simulink model "kinematics_ellipse"  (R2015a)
settings: Solver=ode45  StartTime=0.0  StopTime=500  RelTol=1e-3
libraries: simulink x1
settings Model: Creator=MCLab  LastModifiedBy=MCLab

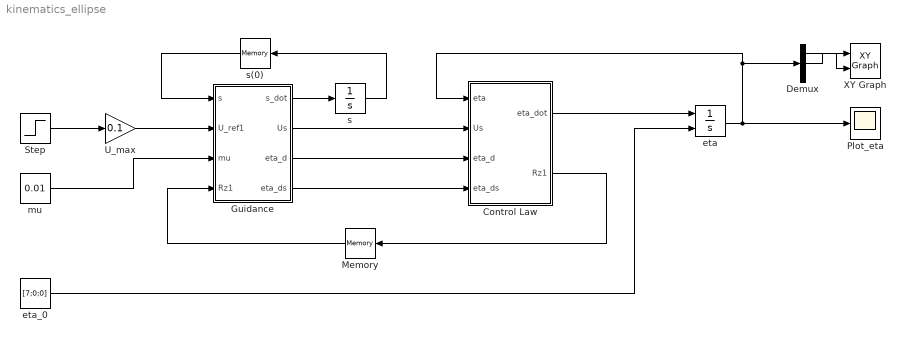
== system kinematics_ellipse ==
  Control Law : MATLAB Function  TreatAsAtomicUnit=on
  Demux : Demux  Outputs=3
  Guidance : MATLAB Function  TreatAsAtomicUnit=on
  Memory : Memory  X0=[0;0;0]
  Plot_eta : Scope
  Step : Step  Time=2000  Before=1  After=-1  SampleTime=0
  U_max : Gain  Gain=0.1
  XY Graph : simulink/Sinks/XY Graph  xmin=-15  xmax=15  ymin=-15  ymax=15  st=-1
  eta : Integrator  InitialConditionSource=external
  eta_0 : Constant  Value=[7;0;0]
  mu : Constant  Value=0.01
  s : Integrator
  s(0) : Memory
  wires:
  Step/1 -> U_max/1
  U_max/1 -> Guidance/2(U_ref1)
  mu/1 -> Guidance/3(mu)
  Guidance/1(s_dot) -> s/1
  s/1 -> s(0)/1
  Guidance/3(eta_d) -> Control Law/3(eta_d)
  Guidance/4(eta_ds) -> Control Law/4(eta_ds)
  Control Law/1(eta_dot) -> eta/1
  eta_0/1 -> eta/2
  Control Law/2(Rz1) -> Memory/1
  Memory/1 -> Guidance/4(Rz1)
  eta/1 -> Plot_eta/1, Control Law/1(eta), Demux/1
  Guidance/2(Us) -> Control Law/2(Us)
  Demux/1 -> XY Graph/2
  Demux/2 -> XY Graph/1
  s(0)/1 -> Guidance/1(s)

== matlab function kinematics_ellipse/Guidance ==
  data: s input; s_dot output; Us output; U_ref1 input; mu input; Rz1 input; eta_d output; eta_ds output
function [s_dot,Us,eta_d,eta_ds] = f(s,U_ref1,mu,Rz1)

%% Ellipse Kinematics

eta_d = [0;0;0];
eta_ds = [0;0;0];

cx = 6;
cy = 0;
rx = 5;
ry = 3;

x_d = cx+rx*cos(s);
y_d = cy+ry*sin(s);

x_ds = -rx*sin(s);
y_ds = ry*cos(s);

x_ds2 = -rx*cos(s);
y_ds2 = -ry*sin(s);

x_ds3 = rx*sin(s);
y_ds3 = -ry*cos(s);

psi_d = atan2(y_ds,x_ds);
psi_ds = (-y_ds*x_ds+x_ds*y_ds2)/(x_ds^2+y_ds^2);
psi_ds2 = ( (-y_ds*x_ds3+x_ds*y_ds3)*(x_ds^2+y_ds^2) - (-y_ds*x_ds2+x_ds*y_ds2)*(2*x_ds2*x_ds+2*y_ds2*y_ds) )/(x_ds^2+y_ds^2)^2;

eta_d = [x_d;y_d;psi_d] ;
eta_ds = [x_ds;y_ds;psi_ds];
eta_ds2 = [x_ds2;y_ds2;psi_ds2];

U_ref2 = U_ref1 ;
Us = U_ref1 / (x_ds^2+y_ds^2)^(1/2);
Us_s = U_ref1 * (x_ds*x_ds2 + y_ds*y_ds2) / (x_ds^2+y_ds^2)^(3/2);


%% Update Law

V1 = - eta_ds'*Rz1 ;
s_dot = Us - mu*V1/norm(eta_ds);


end

== matlab function kinematics_ellipse/Control Law ==
  data: eta input; Us input; eta_d input; eta_ds input; eta_dot output; Rz1 output
function [eta_dot,Rz1] = fcn(eta,Us,eta_d,eta_ds)

psi = 0;
psi = eta(3);
eta_dot = [0;0;0];
nu = [0;0;0];

R = [ cos(psi) , -sin(psi) , 0 ;
      sin(psi) , cos(psi)  , 0 ;
      0            0         1 ] ;

K_p = diag([0.2,0.2,0.1]);

z1 = R'*(eta-eta_d);

Rz1 = R*z1 ;

alpha1 = -K_p*z1 + R'*eta_ds*Us ;

nu = alpha1 ;

eta_dot = R*nu ;

end
